simulink model "untitled"  (R2021a)
settings: Solver=VariableStepAuto  StartTime=0.0  StopTime=10.0  RelTol=1e-3
settings Model: Creator=Name  LastModifiedBy=Name

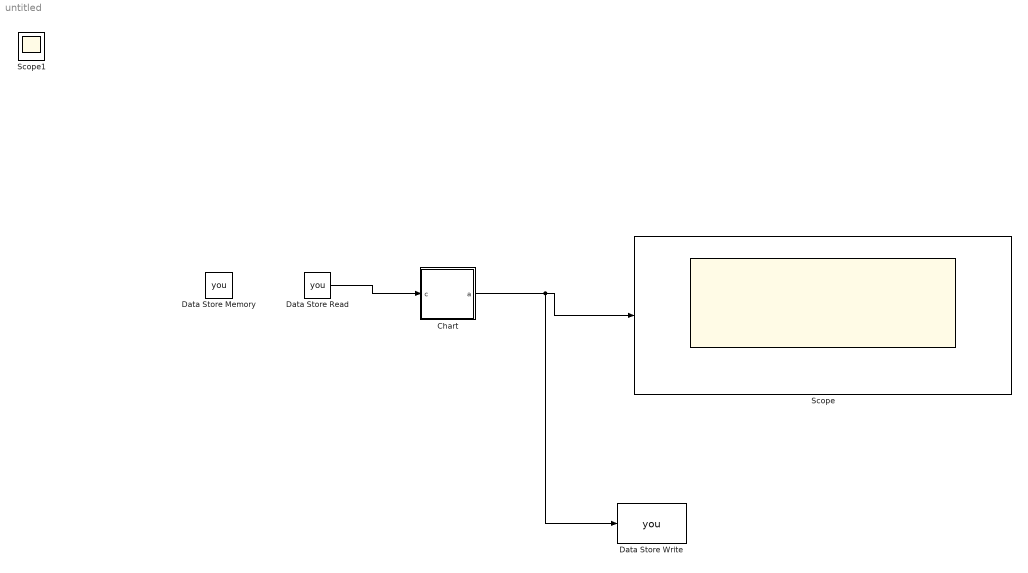
== system untitled ==
  Chart : Stateflow chart  TreatAsAtomicUnit=on
  Data Store Memory : DataStoreMemory  DataStoreName=you  ReadBeforeWriteMsg=warning  WriteAfterWriteMsg=warning  WriteAfterReadMsg=warning  ShareAcrossModelInstances=on  ShowAdditionalParam=off  OutDataTypeStr=double  Dimensions=1
  Data Store Read : DataStoreRead  DataStoreName=you  IndexOptions=Index vector (dialog)  Indices=1  OutputSizes=1
  Data Store Write : DataStoreWrite  DataStoreName=you  IndexOptions=Index vector (dialog)  Indices=1  OutputSizes=1
  Scope : Scope
  Scope1 : Scope
  wires:
  Chart/1(a) -> Data Store Write/1, Scope/1
  Data Store Read/1 -> Chart/1(c)

== stateflow chart untitled/Chart ==
  state stage_1_
    entry:
    a=addf(c);
  (default) -> stage_1_
  data: output function_output size=1; input function_input; a output; c input; you data_store_memory
  function output = addf(input):
    | function output = addf(input)
    | 
    | output=input+1;
    | end
